simulink model "walkingRobotLIPM"  (R2019b)
settings: Solver=ode15s  StartTime=0.0  StopTime=10  EnableMultiTasking=on
PreLoadFcn:
  | robotParameters
  | load('defaultsimulationinputs.mat')
libraries: walkingRobotUtils x2, simulink x1
settings Model: Creator=bkim  LastModifiedBy=scastro
settings DataIOCC: ReturnWorkspaceOutputs=off  OutputSaveName=simout  OutputTimes=0:0.01:10
settings OptimizationCC: LifeSpan=inf
settings DebuggingCC: AllowSymbolicDim=off  PregeneratedLibrarySubsystemCodeDiagnostic=none  SFUnexpectedBacktrackingDiag=warning  SFNoUnconditionalDefaultTransitionDiag=warning  SFExecutionAtInitializationDiag=none  UnitsInconsistencyMsg=none  ArithmeticOperatorsInVariantConditions=warning
settings SFSimCC: SimUseLocalCustomCode=off  CustomCodeUndefinedFunction=UseInterfaceOnly
settings RTWCC: RTWUseLocalCustomCode=off
settings CodeAppCC: StateflowObjectComments=on
settings GRTTargetCC: TargetLangStandard=C89/C90 (ANSI)  GeneratePreprocessorConditionals=Disable all
settings ConfigComp: CovMetricSettings=dw  CovHtmlReporting=on  CovSaveCumulativeToWorkspaceVar=on  CovSaveSingleToWorkspaceVar=on  CovExternalEMLEnable=off  CovSFcnEnable=off
settings SimscapeCC: SimscapeNormalizeSystem=off  SimscapeLogOpenViewer=on  SimscapeLogLimitData=off  SimscapeLogDataHistory=10000
settings ConfigurationSet: Description=SimMechanics 2G
settings DiagnosticsConfigSet: SimMechanicsRigidlyBoundBlock=none
settings ExplorerConfigSet: InternalSimMechanicsExplorerSettings="<ExplorerConfiguration><canonicalview>default</canonicalview><AnimationSetting><BasePlaybackSpeed>1.0</BasePlaybackSpeed><PlaybackSpeedFactor>1.0</PlaybackSpeedFactor></AnimationSetting><TilePanel><TileInfo><Tiles Columns=\"1\" Count=\"1\" Rows=\"1\"><Column Weight=\"1\"/><Row Weight=\"1\"/><Tile Height=\"1\" Width=\"1\" X=\"0\" Y=\"0\"/></Tiles></TileInfo><SceneInfo><SceneViewer><BGColor><R>0.60000002384185791</R><G>0.60000002384185791</G><B>0.60000002384185791</B></BGColor><Camera><DoPerspective>off</DoPerspective><Position><X>-7.93768202680044332</X><Y>23.7533270667132825</Y><Z>3.7574311364824311</Z></Position><Center><X>-0.0429900316406373051</X><Y>-1.53629964608036929</Y><Z>-0.164714621409624673</Z></Center><Up><X>0.0700067588716063866</X><Y>-0.131504315097780378</Y><Z>0.988840567949635152</Z></Up><ViewLimDist>1</ViewLimDist><YLim>2.2322659255588051</YLim><XLim>2.85922950341637039</XLim></Camera></SceneViewer></SceneInfo></TilePanel><MechEditorPanel><Cameras/><GfxPanelCameraMap/><VideoCreator><PlaybackSpeedRatio>1.0</PlaybackSpeedRatio><FrameRate>30</FrameRate><VideoFormat>Motion JPEG AVI</VideoFormat><FrameSize>auto</FrameSize></VideoCreator></MechEditorPanel></ExplorerConfiguration>"

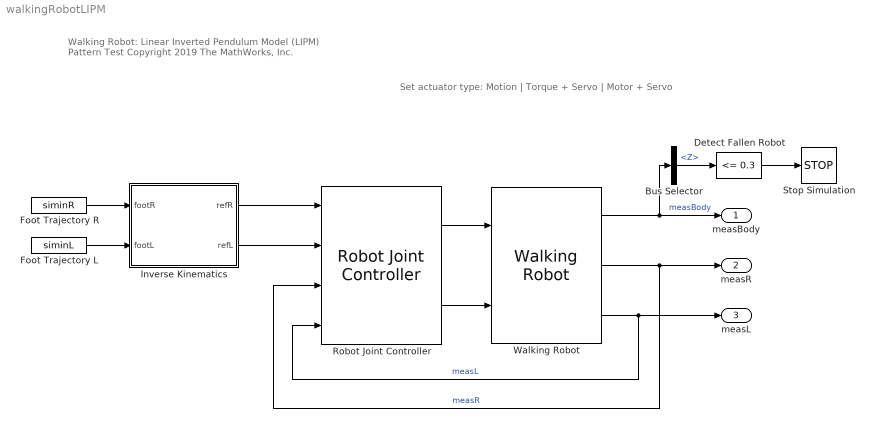
== system walkingRobotLIPM ==
  note: Walking Robot:
      | Linear Inverted Pendulum Model (LIPM) Pattern Test
      |
      | Copyright 2019 The MathWorks, Inc.
  note: Set actuator type:
      | Motion | Torque + Servo | Motor + Servo
  Bus Selector : BusSelector  OutputSignals=Z
  Detect Fallen Robot : simulink/Logic and Bit Operations/Compare To Constant  relop=<=  const=0.3  OutDataTypeStr=boolean
  Foot Trajectory L : FromWorkspace  VariableName=siminL  SampleTime=0  OutputAfterFinalValue=Holding final value
  Foot Trajectory R : FromWorkspace  VariableName=siminR  SampleTime=0  OutputAfterFinalValue=Holding final value
  Inverse Kinematics : Subsystem
  Robot Joint Controller : walkingRobotUtils/Robot Joint Controller  SystemSampleTime=-1  Latency=0  AutoFrameSizeCalculation=off
  Stop Simulation : Stop
  Walking Robot : walkingRobotUtils/Walking Robot  SystemSampleTime=-1  Latency=0  AutoFrameSizeCalculation=off
  measBody : Outport  VectorParamsAs1DForOutWhenUnconnected=off
  measR : Outport  Port=2  VectorParamsAs1DForOutWhenUnconnected=off
  measL : Outport  Port=3  VectorParamsAs1DForOutWhenUnconnected=off
  wires:
  Robot Joint Controller/1 -> Walking Robot/1
  Walking Robot/3 -> Robot Joint Controller/4, measL/1  "measL"
  Walking Robot/2 -> Robot Joint Controller/3, measR/1  "measR"
  Inverse Kinematics/1(refR) -> Robot Joint Controller/1
  Inverse Kinematics/2(refL) -> Robot Joint Controller/2
  Detect Fallen Robot/1 -> Stop Simulation/1
  Walking Robot/1 -> Bus Selector/1, measBody/1  "measBody"
  Foot Trajectory L/1 -> Inverse Kinematics/2(footL)
  Robot Joint Controller/2 -> Walking Robot/2
  Foot Trajectory R/1 -> Inverse Kinematics/1(footR)
  Bus Selector/1 -> Detect Fallen Robot/1  "<Z>"

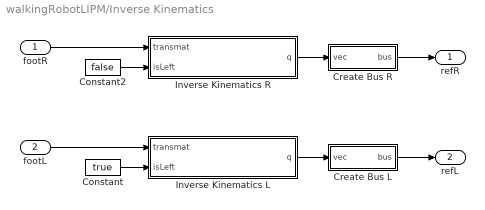
== system walkingRobotLIPM/Inverse Kinematics ==
  footR : Inport
  footL : Inport  Port=2
  Constant : Constant  Value=true
  Constant2 : Constant  Value=false
  Create Bus L : Subsystem
  Create Bus R : Subsystem
  Inverse Kinematics L : MATLAB Function  TreatAsAtomicUnit=on
  Inverse Kinematics R : MATLAB Function  TreatAsAtomicUnit=on
  refR : Outport
  refL : Outport  Port=2
  wires:
  footR/1 -> Inverse Kinematics R/1(transmat)
  Inverse Kinematics L/1(q) -> Create Bus L/1(vec)
  Constant2/1 -> Inverse Kinematics R/2(isLeft)
  Create Bus R/1(bus) -> refR/1
  Create Bus L/1(bus) -> refL/1
  Constant/1 -> Inverse Kinematics L/2(isLeft)
  Inverse Kinematics R/1(q) -> Create Bus R/1(vec)
  footL/1 -> Inverse Kinematics L/1(transmat)

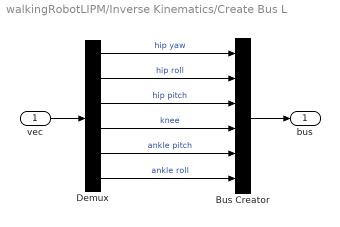
== system walkingRobotLIPM/Inverse Kinematics/Create Bus L ==
  vec : Inport
  Bus Creator : BusCreator  Inputs=6
  Demux : Demux  Outputs=6
  bus : Outport  VectorParamsAs1DForOutWhenUnconnected=off
  wires:
  Bus Creator/1 -> bus/1
  vec/1 -> Demux/1
  Demux/6 -> Bus Creator/6  "ankle roll"
  Demux/4 -> Bus Creator/4  "knee"
  Demux/2 -> Bus Creator/2  "hip roll"
  Demux/5 -> Bus Creator/5  "ankle pitch"
  Demux/1 -> Bus Creator/1  "hip yaw"
  Demux/3 -> Bus Creator/3  "hip pitch"

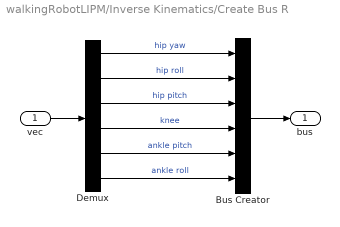
== system walkingRobotLIPM/Inverse Kinematics/Create Bus R ==
  vec : Inport
  Bus Creator : BusCreator  Inputs=6
  Demux : Demux  Outputs=6
  bus : Outport  VectorParamsAs1DForOutWhenUnconnected=off
  wires:
  Demux/3 -> Bus Creator/3  "hip pitch"
  Demux/1 -> Bus Creator/1  "hip yaw"
  Demux/5 -> Bus Creator/5  "ankle pitch"
  Demux/2 -> Bus Creator/2  "hip roll"
  Demux/4 -> Bus Creator/4  "knee"
  Demux/6 -> Bus Creator/6  "ankle roll"
  vec/1 -> Demux/1
  Bus Creator/1 -> bus/1

== matlab function walkingRobotLIPM/Inverse Kinematics/Inverse Kinematics L ==
  data: transmat input; q output; isLeft input
function q = inverseKinematics(transmat, isLeft)
q = invKinBody2Foot(transmat, isLeft);

== matlab function walkingRobotLIPM/Inverse Kinematics/Inverse Kinematics R ==
  data: transmat input; q output; isLeft input
function q = inverseKinematics(transmat, isLeft)
q = invKinBody2Foot(transmat, isLeft);
